simulink model "ESTS_TFY_LatForceFromFx_test"  (R2023b)
settings: Solver=VariableStepAuto  StartTime=0.0  StopTime=10.0  RelTol=1e-3
libraries: ESTS_TFY_LatForceFromFx x1
settings Model: Creator=blatak  LastModifiedBy=blatak

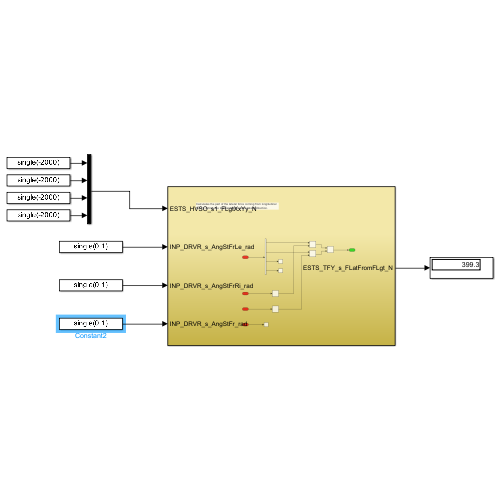
[thumbnail: Simulink's stored preview of the top-level diagram]
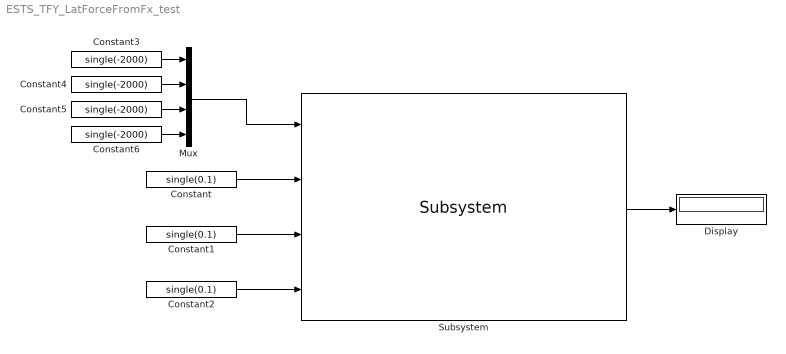
== system ESTS_TFY_LatForceFromFx_test ==
  Constant : Constant  Value=single(0.1)
  Constant1 : Constant  Value=single(0.1)
  Constant2 : Constant  Value=single(0.1)
  Constant{3..6} (4 alike) : Constant  Value=single(-2000)
  Display : Display
  Mux : Mux
  Subsystem : ESTS_TFY_LatForceFromFx/Subsystem  SystemSampleTime=-1  VariantActivationTime=update diagram  AllowFlexibleInterface=on  Latency=0  AutoFrameSizeCalculation=off
  wires:
  Constant/1 -> Subsystem/2
  Constant1/1 -> Subsystem/3
  Constant2/1 -> Subsystem/4
  Constant3/1 -> Mux/1
  Constant4/1 -> Mux/2
  Constant6/1 -> Mux/4
  Constant5/1 -> Mux/3
  Subsystem/1 -> Display/1
  Mux/1 -> Subsystem/1
